simulink library "tqd"  (R2021b)
settings: Solver=VariableStepAuto  StartTime=0.0  StopTime=10.0  RelTol=1e-3
undefined symbols (not defined in the file): ATQD_AfterTqMinGain_X_Deg, ATQD_APSCreepBaseTqD_X_kph, ATQD_APSCreepBaseTqD_Y_Deg, ATQD_APSCreepBaseTqR_X_kph, ATQD_APSCreepBaseTqR_Y_Deg, ATQD_APSCreepIterm_X_kph, ATQD_APSCreepIterm_Y_kph, ATQD_APSCreepPterm_X_kph, ATQD_APSCreepPterm_Y_kph, ATQD_APSDecReq_X_kph, ATQD_APSDecReq_Y_mps2, ATQD_APSDecReqCMD_X_kph, ATQD_APSDecReqTs_X_pct, ATQD_APSDecTimeGain_X_Deg, ATQD_APSDecTimeGain_Y_s, ATQD_APSReqLowSpd_X_Deg, ATQD_AutoHoldReleaseBPS_X_Deg, ATQD_AWDLoadTrqnsGain_X_kg, ATQD_AWDLoadTrqnsGain_Y_pct, ATQD_BOSEnBPSPosn_X_kph, ATQD_BOSMap_X_rpm, ATQD_BOSMap_Y_pct, ATQD_CreepBaseTqD_X_kph, ATQD_CreepBaseTqD_Y_Deg, ATQD_CreepBaseTqR_X_kph, ATQD_CreepBaseTqR_Y_Deg, ATQD_CreepBPSDisPosn_X_Deg, ATQD_CreepBPSDisPosnR_X_Deg, ATQD_CreepBPSEnPosn_X_Deg, ATQD_CreepBPSEnPosnR_X_Deg, ATQD_CreepDeltaTq_X_kph, ATQD_CreepIterm_X_kph, ATQD_CreepIterm_Y_kph, ATQD_CreepItermMaxLimit_X_pct, ATQD_CreepPreloadTime_X_kph, ATQD_CreepPreloadTq_X_kph, ATQD_CreepPreloadTq_Y_s, ATQD_CreepProtTq_X_Deg, ATQD_CreepPterm_X_kph, ATQD_CreepPterm_Y_kph, ATQD_CreepRrTqSpRat_X_rpm, ATQD_CreepRrTqSpRat_Y_Nm, ATQD_CreepTargetSpdD_X_pct, ATQD_CreepTargetSpdR_X_pct, ATQD_ECOTqMapD_X_rpm, ATQD_ECOTqMapD_Y_pct, ATQD_EMTqMapD_X_rpm, ATQD_EMTqMapD_Y_pct, ATQD_EOPDTqMapDCon_X_rpm, ATQD_EOPDTqMapDCon_Y_Deg, ATQD_EscapeModePedTq_X_pct, ATQD_EscapeModePedTq_Y_rpm, ATQD_EscapeModePedTqFr_X_pct, ATQD_EscapeModePedTqFr_Y_rpm, ATQD_EstInitVehWeight_X_c, ATQD_FAfterTqCMDGain_X_rpm, ATQD_FAfterTqCMDGain_Y_pct, ATQD_FrLossMAPLowV_X_rpm, ATQD_FrLossMAPLowV_Y_Nm, ATQD_FrMotActReduce_X_rpm ... (+772)
libraries: simulink x211, hcu_lib x179, tqr x3
(part 1 of 28)
settings Model: Creator=13615  LastModifiedBy=FVT24123
settings SolverCC: AlgebraicLoopSolver=TrustRegion
settings DataIOCC: SaveFormat=Array  SignalLoggingSaveFormat=ModelDataLogs  ReturnWorkspaceOutputs=off
settings OptimizationCC: BlockReduction=off  BooleanDataType=off
settings DebuggingCC: SaveWithParameterizedLinksMsg=none  UnderspecifiedInitializationDetection=Classic  MergeDetectMultiDrivingBlocksExec=none  SignalResolutionControl=TryResolveAllWithWarning
settings HardwareCC: TargetUnknown=on
settings ModelReferenceCC: PropagateSignalLabelsOutOfModel=off
settings SFSimCC: SimUseLocalCustomCode=off
settings RTWCC: RTWUseLocalCustomCode=off
settings ConfigComp: CovMetricSettings=dw  CovSaveCumulativeToWorkspaceVar=on  CovSaveSingleToWorkspaceVar=on

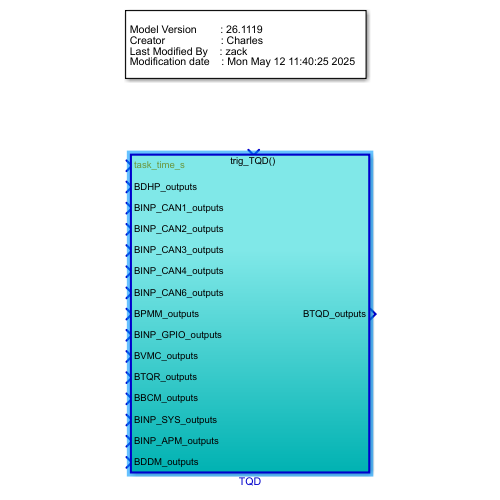
[thumbnail: Simulink's stored preview of the top-level diagram]
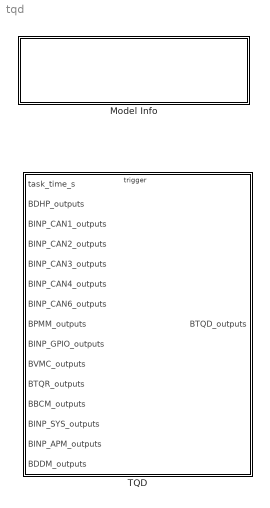
== system tqd ==
  Model Info : Subsystem  LoadFcn=slcm LoadBlock;  InitFcn=slcm('UpdateAllCMBlocksInThisModelInit')  mask(CMBlock){InitialSaveTempField=, InitialBlockCM=None, BlockCM=None, Frame=on, SaveTempField=, DisplayStringWithTags=|, MaskDisplayString=Model Version        : 26.1294\nCreator                   : Charles\nLast Modified By    : FVT24123\nModification date    : Mon Sep 22 17:25:36 2025, HorizontalTextAlignment=Left, LeftAlignmentValue=0.02, SourceBlockDiagram=tqd, TagMaxNumber=20, CMTag1=, CMTag2=, CMTag3=, CMTag4=, CMTag5=, CMTag6=, CMTag7=, CMTag8=, CMTag9=, CMTag10=, CMTag11=, CMTag12=, CMTag13=, CMTag14=, CMTag15=, CMTag16=, CMTag17=, CMTag18=, CMTag19=, CMTag20=}
      mask DisplayStringWithTags=|
      | Model Version        : %<ModelVersion>
      | Creator                   : Charles
      | Last Modified By    : %<LastModifiedBy>
      | Modification date    : %<LastModificationDate>
      mask help: This block allows revision control information to be displayed within the model.
      settings: CopyFcn=slcm CopyBlock;  DeleteFcn=slcm Cancel;  PostSaveFcn=slcm('UpdateAllCMBlocksInThisModel')  NameChangeFcn=slcm Rename;  OpenFcn=slcm
      mask Display: text(str2num(LeftAlignmentValue), 0.5, MaskDisplayString, 'HorizontalAlignment', HorizontalTextAlignment)
  TQD : Subsystem
      settings: RTWSystemCode=Nonreusable function  RTWFcnNameOpts=Use subsystem name  RTWFileNameOpts=Use subsystem name

== system tqd/Model Info ==
  EmptySubsystem : Subsystem

== system tqd/TQD ==
  task_time_s : Inport
  BDHP_outputs : Inport  Port=2  OutDataTypeStr=Bus: BDHP_outputs
  BINP_CAN1_outputs : Inport  Port=3  OutDataTypeStr=Bus: BINP_CAN1_outputs
  BINP_CAN2_outputs : Inport  Port=4  OutDataTypeStr=Bus: BINP_CAN2_outputs
  BINP_CAN3_outputs : Inport  Port=5  OutDataTypeStr=Bus: BINP_CAN3_outputs
  BINP_CAN4_outputs : Inport  Port=6  OutDataTypeStr=Bus: BINP_CAN4_outputs
  BINP_CAN6_outputs : Inport  Port=7  OutDataTypeStr=Bus: BINP_CAN6_outputs
  BPMM_outputs : Inport  Port=8  OutDataTypeStr=Bus: BPMM_outputs
  BINP_GPIO_outputs : Inport  Port=9  OutDataTypeStr=Bus: BINP_GPIO_outputs
  BVMC_outputs : Inport  Port=10  OutDataTypeStr=Bus: BVMC_outputs
  BTQR_outputs : Inport  Port=11  OutDataTypeStr=Bus: BTQR_outputs  LockScale=on
  BBCM_outputs : Inport  Port=12  OutDataTypeStr=Bus: BBCM_outputs
  BINP_SYS_outputs : Inport  Port=13  OutDataTypeStr=Bus: BINP_SYS_outputs
  BINP_APM_outputs : Inport  Port=14  OutDataTypeStr=Bus: BINP_APM_outputs
  BDDM_outputs : Inport  Port=15  OutDataTypeStr=Bus: BDDM_outputs
  trig_TQD : TriggerPort  TriggerType=function-call  VariantControl=(inherit)
  Bus Creator1 : BusCreator  Inputs=118  OutDataTypeStr=Bus: BTQD_outputs  NonVirtualBus=on
  Bus Selector : BusSelector  OutputSignals=VINP_IVIPWModeReq_enum,VINP_IVICreepSWReq_flg,VINP_RollModeSWCmd_enum,VINP_IVIPwrLockSW_enum,VINP_IVIISAOffsetSpd_enum,VINP_Distanceunit_flg,VINP_SmartEcoModeSW_flg,VINP_IVISnowModeCmd_flg,VINP_IVIACCAdaptiveSta_flg,VINP_IVITrailerModeSWSta_flg
  Bus Selector1 : BusSelector  OutputSignals=VDHP_ActAPSPosn_pct,VDHP_LowIdleAccPedal_flg
  Bus Selector10 : BusSelector  OutputSignals=VBCM_BrakeLamp_flg,VBCM_UserNow_enum
  Bus Selector11 : BusSelector  OutputSignals=VINP_FlashRegenMode_enum,VINP_VehicleType_enum,VINP_SWCType_enum
  Bus Selector12 : BusSelector  OutputSignals=VINP_CAASSta_enum,VINP_APSStaSystem_enum
  Bus Selector13 : BusSelector  OutputSignals=VINP_FrEDURotateDirction_enum,VINP_RrEDURotateDirction_enum,VINP_FrTMSpd_rpm,VINP_RrTMSpd_rpm,VINP_FrRegenAvailTq_Nm,VINP_RrRegenAvailTq_Nm,VINP_FrEDURealTMTq_Nm,VINP_RrEDURealTMTq_Nm,VINP_FrMotorAvailTq_Nm,VINP_RrMotorAvailTq_Nm,VINP_MCUWarnF_enum,VINP_MCUWarnR_enum,VINP_FrMCUDCBusVolt_V,VINP_RrMCUDCBusVolt_V,VINP_FrMCUTemp_C,VINP_FrTMTemp_C,VINP_RrMCUTemp_C,VINP_RrTMTemp_C
  Bus Selector14 : BusSelector  OutputSignals=VINP_SWCRegenUp_flg,VINP_SWCRegenDown_flg
  Bus Selector15 : BusSelector  OutputSignals=VDDM_VCURAPSErrLv2_flg,VDDM_VCURAPSErrLv3_flg,VDDM_EPBSigErrCFS_flg,VDDM_EPB1Err_flg,VDDM_ESC1Err_flg,VDDM_ESC5Err_flg,VDDM_LimpHomeAct_flg,VDDM_VehMalfunLevel_enum,VDDM_Shifter1Err_flg,VDDM_ShifterSigErrCFS_flg,VDDM_MCUF1Err_flg,VDDM_MCUR1Err_flg,VDDM_RegenErrCFS_flg,VDDM_4D2CErr_flg
  Bus Selector2 : BusSelector  OutputSignals=VINP_VehSpeed_kph,VINP_BrkSwSta_flg,VINP_BrkSwV_flg,VINP_BrkPedalPos_pct,VINP_BrkPedalPosSta_flg,VINP_FrPTCSActive_flg,VINP_RrPTCSActive_flg,VINP_FrntAxlTrqReqDrv_Nm,VINP_RearAxlTrqReqDrv_Nm,VINP_FrRBCActive_flg,VINP_RrRBCActive_flg,VINP_FrntAxlTrqReqBrk_Nm,VINP_RearAxlTrqReqBrk_Nm,VINP_CrashOutputSts_enum,VINP_LongAccel_Gps,VINP_EPBCarWashMode_flg,VINP_EPBErrSta_enum,VINP_EPBSta_enum,VINP_DOASta_flg,VINP_GRADE_Deg,VINP_HSAActive_flg,VINP_DriverSeatBeltCmd_flg,VINP_AVHActive_flg,VINP_PsngrSeatBeltCmd_flg,VINP_RDriverSeatBeltCmd_flg,VINP_RCenterSeatBeltCmd_flg,VINP_RPsngrSeatBeltCmd_flg,VINP_YawRate_degps,VINP_SASAngle_Deg,VINP_ESCActive_flg,VINP_ABSActive_flg,VINP_LFRawWhlSpeed_kph,VINP_LRRawWhlSpeed_kph,VINP_RFRawWhlSpeed_kph,VINP_RRRawWhlSpeed_kph,VINP_ESCOFFStatus_enum
  Bus Selector3 : BusSelector  OutputSignals=VINP_BrakeSWGPIO_flg,VINP_CrashSignalGPIO_flg,VINP_DrDoorSW_flg,VINP_SeatSW_flg,VINP_HoodSW_flg,VINP_TailgateSW_flg,VINP_PsDoorSW_flg,VINP_RRDoorSW_flg,VINP_RLDoorSW_flg
  Bus Selector4 : BusSelector  OutputSignals=VINP_ShifterHandleCmd_enum,VINP_HVBPwrAvailDchrg_kW,VINP_HVBPwrAvailChrg_kW,VINP_HVBattErr_flg,VINP_DCDCFaultSta_enum,VINP_ChrgPlugSta_enum,VINP_HVBattSOC_pct,VINP_HVBattSOCDis_pct,VINP_HVBMTempMax_C,VINP_HVBMTempMin_C,VINP_ShifterFailsta_enum
  Bus Selector5 : BusSelector  OutputSignals=VVMC_ADASForceIdle_flg,VVMC_ACCRequiredAccel_mps2,VVMC_ACCVehHoldReq_flg,VVMC_ADASActive_flg,VVMC_ADASWhlTqReq_Nm,VVMC_CruzActive_flg,VVMC_CruzWhlTqReq_Nm,VVMC_MSAActive_flg,VVMC_MSAWhlTqReq_Nm,VVMC_APSActive_flg,VVMC_APSSpeedCMD_kph,VVMC_APSShiftPosnReq_enum,VVMC_ACCPedalOvrd_flg,VVMC_LongAcc_Gps,VVMC_ActMaxSlideRate_pct,VVMC_EstSlope_Deg,VVMC_APSReq_enum,VVMC_RWDRDCActive_enum,VVMC_ActLRSlideRate_pct,VVMC_ActRRSlideRate_pct,VVMC_ActStESCYaw_Dps,VVMC_CCCtrlSta_enum,VVMC_MSACtrlSta_enum,VVMC_LVDAACCStatusInformation_flg,VVMC_ACCObjDist_m,VVMC_MeterIndSpeed_raw32,VVMC_RearTqRatio_rat,VVMC_CalibratedGyroY_Dps,VVMC_CAASActive_flg,VVMC_SetACCDisableAPS_flg
  Bus Selector6 : BusSelector  OutputSignals=VINP_SWCResUpSta_flg,VINP_SWCSetdownSta_flg,VINP_SWCACCSta_flg,VINP_SWCCANCELSta_flg,VINP_SWC2LScrollUpSta_flg,VINP_SWC2LScrollDownSta_flg,VINP_SWC2LScrollPressSta_flg,VINP_SWC2LADASSta_flg,VINP_SWC2RScrollPressSta_flg,VINP_SWC2RScrollUpSta_flg,VINP_SWC2RScrollDownSta_flg,VINP_SWC2LDriveModeSta_flg,VINP_SWC2RRightSta_flg,VINP_SWC2RLeftSta_flg,VINP_SWC2RCustomizeSta_flg
  Bus Selector7 : BusSelector  OutputSignals=VPMM_PowerSta_enum,VPMM_DrivetrainSelect_enum,VPMM_SysPowerMode_enum
  Bus Selector8 : BusSelector  OutputSignals=VTQR_ActualFEDUWhlTqReq_Nm,VTQR_ActualREDUWhlTqReq_Nm,VTQR_NoABSFEDUWhlTqReq_Nm,VTQR_NoABSREDUWhlTqReq_Nm,VTQR_RShaftSpdTqLimLow_flg,VTQR_RTimerTqLimLow_flg,VTQR_FShaftSpdTqLimLow_flg,VTQR_FTimerTqLimLow_flg,VTQR_FrFirstOrderInpTs_c,VTQR_RrFirstOrderInpTs_c,VTQR_FrRateLimitInc_Nm,VTQR_FrRateLimitDec_Nm,VTQR_RrRateLimitInc_Nm,VTQR_RrRateLimitDec_Nm,VTQR_FrTqZeroTransLowBound_Nm,VTQR_RrTqZeroTransUpBound_Nm
  Bus Selector9 : BusSelector  OutputSignals=VINP_ADASISASta_enum,VINP_ADASVehSpdLim_enum,VINP_ADASACCSta_enum,VINP_ADASSLIFSpdLim_enum,VINP_ADASAEBSta_enum
  Constant2 : Constant  Value=KTQD_IVIEscapeModeCmd_flg
  Constant4 : Constant  Value=KTQD_BCMUserNowSetting_enum
  Ground1 : Ground
  SWC_HandShake : Subsystem
  Subsystem : Subsystem
  TorqueDemand : Subsystem
  BTQD_outputs : Outport  OutDataTypeStr=Bus: BTQD_outputs
  wires:
  Bus Selector2/19 -> TorqueDemand/25(VINP_DOASta_flg)  "<VINP_DOASta_flg>"
  Bus Selector2/18 -> TorqueDemand/24(VINP_EPBSta_enum)  "<VINP_EPBSta_enum>"
  Bus Selector2/17 -> TorqueDemand/23(VINP_EPBErrSta_enum)  "<VINP_EPBErrSta_enum>"
  Bus Selector2/16 -> TorqueDemand/22(VINP_EPBCarWashMode_flg)  "<VINP_EPBCarWashMode_flg>"
  Bus Selector8/2 -> TorqueDemand/139(VTQR_ActualREDUWhlTqReq_Nm)  "<VTQR_ActualREDUWhlTqReq_Nm>"
  Bus Selector2/15 -> TorqueDemand/21(VINP_LongAccel_Gps)  "<VINP_LongAccel_Gps>"
  Bus Selector8/1 -> TorqueDemand/138(VTQR_ActualFEDUWhlTqReq_Nm)  "<VTQR_ActualFEDUWhlTqReq_Nm>"
  Bus Selector5/6 -> TorqueDemand/104(VVMC_CruzActive_flg)  "<VVMC_CruzActive_flg>"
  BTQR_outputs/1 -> Bus Selector8/1
  Bus Selector3/2 -> TorqueDemand/130(VINP_CrashSignalGPIO_flg)  "<VINP_CrashSignalGPIO_flg>"
  Bus Selector3/1 -> TorqueDemand/129(VINP_BrakeSWGPIO_flg)  "<VINP_BrakeSWGPIO_flg>"
  Bus Selector5/9 -> TorqueDemand/107(VVMC_MSAWhlTqReq_Nm)  "<VVMC_MSAWhlTqReq_Nm>"
  Bus Selector5/4 -> TorqueDemand/102(VVMC_ADASActive_flg)  "<VVMC_ADASActive_flg>"
  Bus Selector5/8 -> TorqueDemand/106(VVMC_MSAActive_flg)  "<VVMC_MSAActive_flg>"
  Bus Selector5/7 -> TorqueDemand/105(VVMC_CruzWhlTqReq_Nm)  "<VVMC_CruzWhlTqReq_Nm>"
  Bus Selector5/5 -> TorqueDemand/103(VVMC_ADASWhlTqReq_Nm)  "<VVMC_ADASWhlTqReq_Nm>"
  Bus Selector2/14 -> TorqueDemand/20(VINP_CrashOutputSts_enum)  "<VINP_CrashOutputSts_enum>"
  BDHP_outputs/1 -> Bus Selector1/1
  Bus Selector2/5 -> TorqueDemand/11(VINP_BrkPedalPosSta_flg)  "<VINP_BrkPedalPosSta_flg>"
  Bus Selector/1 -> TorqueDemand/43(VINP_IVIPWModeReq_enum)  "<VINP_IVIPWModeReq_enum>"
  [BINP_CAN4_outputs] -> Bus Selector6/1  "BINP_CAN4_outputs"
  BINP_CAN2_outputs/1 -> Bus Selector/1  "BINP_CAN2_outputs"
  Ground1/1 -> TorqueDemand/154(VINP_PBWMotorPos_enum)
  BVMC_outputs/1 -> Bus Selector5/1
  Bus Selector2/11 -> TorqueDemand/17(VINP_RrRBCActive_flg)  "<VINP_RrRBCActive_flg>"
  Bus Selector2/7 -> TorqueDemand/13(VINP_RrPTCSActive_flg)  "<VINP_RrPTCSActive_flg>"
  Bus Selector7/2 -> TorqueDemand/5(VPMM_DrivetrainSelect_enum)  "<VPMM_DrivetrainSelect_enum>"
  BINP_GPIO_outputs/1 -> Bus Selector3/1
  Bus Selector1/2 -> TorqueDemand/3(VDHP_LowIdleAccPedal_flg)  "<VDHP_LowIdleAccPedal_flg>"
  Bus Selector1/1 -> TorqueDemand/2(VDHP_ActAPSPosn_pct)  "<VDHP_ActAPSPosn_pct>"
  Bus Selector2/10 -> TorqueDemand/16(VINP_FrRBCActive_flg)  "<VINP_FrRBCActive_flg>"
  Bus Selector2/9 -> TorqueDemand/15(VINP_RearAxlTrqReqDrv_Nm)  "<VINP_RearAxlTrqReqDrv_Nm>"
  Bus Selector2/8 -> TorqueDemand/14(VINP_FrntAxlTrqReqDrv_Nm)  "<VINP_FrntAxlTrqReqDrv_Nm>"
  Bus Selector2/13 -> TorqueDemand/19(VINP_RearAxlTrqReqBrk_Nm)  "<VINP_RearAxlTrqReqBrk_Nm>"
  Bus Selector2/12 -> TorqueDemand/18(VINP_FrntAxlTrqReqBrk_Nm)  "<VINP_FrntAxlTrqReqBrk_Nm>"
  Bus Selector2/4 -> TorqueDemand/10(VINP_BrkPedalPos_pct)  "<VINP_BrkPedalPos_pct>"
  Bus Selector2/3 -> TorqueDemand/9(VINP_BrkSwV_flg)  "<VINP_BrkSwV_flg>"
  Bus Selector2/2 -> TorqueDemand/8(VINP_BrkSwSta_flg)  "<VINP_BrkSwSta_flg>"
  Bus Selector2/1 -> TorqueDemand/7(VINP_VehSpeed_kph)  "<VINP_VehSpeed_kph>"
  Bus Selector2/6 -> TorqueDemand/12(VINP_FrPTCSActive_flg)  "<VINP_FrPTCSActive_flg>"
  Bus Selector7/1 -> TorqueDemand/4(VPMM_PowerSta_enum)  "<VPMM_PowerSta_enum>"
  task_time_s/1 -> TorqueDemand/1(task_time_s)  "task_time_s"
  BINP_CAN1_outputs/1 -> Bus Selector2/1
  BPMM_outputs/1 -> Bus Selector7/1
  Bus Creator1/1 -> BTQD_outputs/1  "BTQD_outputs"
  Bus Selector2/20 -> TorqueDemand/26(VINP_GRADE_Deg)  "<VINP_GRADE_Deg>"
  Bus Selector2/21 -> TorqueDemand/27(VINP_HSAActive_flg)  "<VINP_HSAActive_flg>"
  Bus Selector/2 -> TorqueDemand/44(VINP_IVICreepSWReq_flg)  "<VINP_IVICreepSWReq_flg>"
  Bus Selector2/22 -> TorqueDemand/28(VINP_DriverSeatBeltCmd_flg)  "<VINP_DriverSeatBeltCmd_flg>"
  Bus Selector3/3 -> TorqueDemand/131(VINP_DrDoorSW_flg)  "<VINP_DrDoorSW_flg>"
  Bus Selector3/4 -> TorqueDemand/132(VINP_SeatSW_flg)  "<VINP_SeatSW_flg>"
  Bus Selector7/3 -> TorqueDemand/6(VPMM_SysPowerMode_enum)  "<VPMM_SysPowerMode_enum>"
  Bus Selector8/3 -> TorqueDemand/140(VTQR_NoABSFEDUWhlTqReq_Nm)  "<VTQR_NoABSFEDUWhlTqReq_Nm>"
  Bus Selector8/4 -> TorqueDemand/141(VTQR_NoABSREDUWhlTqReq_Nm)  "<VTQR_NoABSREDUWhlTqReq_Nm>"
  Bus Selector2/23 -> TorqueDemand/29(VINP_AVHActive_flg)  "<VINP_AVHActive_flg>"
  Bus Selector5/10 -> TorqueDemand/108(VVMC_APSActive_flg)  "<VVMC_APSActive_flg>"
  Bus Selector5/11 -> TorqueDemand/109(VVMC_APSSpeedCMD_kph)  "<VVMC_APSSpeedCMD_kph>"
  Bus Selector5/12 -> TorqueDemand/110(VVMC_APSShiftPosnReq_enum)  "<VVMC_APSShiftPosnReq_enum>"
  Bus Selector5/13 -> TorqueDemand/111(VVMC_ACCPedalOvrd_flg)  "<VVMC_ACCPedalOvrd_flg>"
  Bus Selector2/24 -> TorqueDemand/30(VINP_PsngrSeatBeltCmd_flg)  "<VINP_PsngrSeatBeltCmd_flg>"
  Bus Selector2/25 -> TorqueDemand/31(VINP_RDriverSeatBeltCmd_flg)  "<VINP_RDriverSeatBeltCmd_flg>"
  Bus Selector2/27 -> TorqueDemand/33(VINP_RPsngrSeatBeltCmd_flg)  "<VINP_RPsngrSeatBeltCmd_flg>"
  Bus Selector/3 -> TorqueDemand/45(VINP_RollModeSWCmd_enum)  "<VINP_RollModeSWCmd_enum>"
  Bus Selector5/14 -> TorqueDemand/112(VVMC_LongAcc_Gps)  "<VVMC_LongAcc_Gps>"
  Bus Selector5/15 -> TorqueDemand/113(VVMC_ActMaxSlideRate_pct)  "<VVMC_ActMaxSlideRate_pct>"
  Bus Selector5/17 -> TorqueDemand/115(VVMC_APSReq_enum)  "<VVMC_APSReq_enum>"
  Bus Selector5/16 -> TorqueDemand/114(VVMC_EstSlope_Deg)  "<VVMC_EstSlope_Deg>"
  Bus Selector2/26 -> TorqueDemand/32(VINP_RCenterSeatBeltCmd_flg)  "<VINP_RCenterSeatBeltCmd_flg>"
  Bus Selector3/5 -> TorqueDemand/133(VINP_HoodSW_flg)  "<VINP_HoodSW_flg>"
  Bus Selector3/6 -> TorqueDemand/134(VINP_TailgateSW_flg)  "<VINP_TailgateSW_flg>"
  Bus Selector3/7 -> TorqueDemand/135(VINP_PsDoorSW_flg)  "<VINP_PsDoorSW_flg>"
  Bus Selector3/8 -> TorqueDemand/136(VINP_RRDoorSW_flg)  "<VINP_RRDoorSW_flg>"
  Bus Selector3/9 -> TorqueDemand/137(VINP_RLDoorSW_flg)  "<VINP_RLDoorSW_flg>"
  Bus Selector6/1 -> TorqueDemand/82(VINP_SWCResUpSta_flg)  "<VINP_SWCResUpSta_flg>"
  Bus Selector/4 -> TorqueDemand/46(VINP_IVIPwrLockSW_enum)  "<VINP_IVIPwrLockSW_enum>"
  Bus Selector5/18 -> TorqueDemand/116(VVMC_RWDRDCActive_enum)  "<VVMC_RWDRDCActive_enum>"
  Bus Selector5/19 -> TorqueDemand/117(VVMC_ActLRSlideRate_pct)  "<VVMC_ActLRSlideRate_pct>"
  Bus Selector5/20 -> TorqueDemand/118(VVMC_ActRRSlideRate_pct)  "<VVMC_ActRRSlideRate_pct>"
  Bus Selector5/21 -> TorqueDemand/119(VVMC_ActStESCYaw_degps)  "<VVMC_ActStESCYaw_Dps>"
  Bus Selector2/28 -> TorqueDemand/34(VINP_YawRate_degps)  "<VINP_YawRate_degps>"
  Bus Selector2/29 -> TorqueDemand/35(VINP_SASAngle_Deg)  "<VINP_SASAngle_Deg>"
  TorqueDemand/24(VTQD_DriverWhlTqDemRr_Nm) -> Bus Creator1/24
  TorqueDemand/25(VTQD_FrEDUActTq_Nm) -> Bus Creator1/25
  TorqueDemand/26(VTQD_RrEDUActTq_Nm) -> Bus Creator1/26
  TorqueDemand/27(VTQD_FrEDURolRgnTq_Nm) -> Bus Creator1/27
  TorqueDemand/28(VTQD_RrEDURolRgnTq_Nm) -> Bus Creator1/28
  TorqueDemand/29(VTQD_FrEDUSpd_rpm) -> Bus Creator1/29
  TorqueDemand/30(VTQD_RrEDUSpd_rpm) -> Bus Creator1/30
  TorqueDemand/42(VTQD_FrUdcMin_V) -> Bus Creator1/42
  TorqueDemand/43(VTQD_FrUdcMax_V) -> Bus Creator1/43
  TorqueDemand/44(VTQD_RrIdcMin_A) -> Bus Creator1/44
  TorqueDemand/45(VTQD_RrIdcMax_A) -> Bus Creator1/45
  TorqueDemand/46(VTQD_RrUdcMin_V) -> Bus Creator1/46
  TorqueDemand/47(VTQD_RrUdcMax_V) -> Bus Creator1/47
  TorqueDemand/48(VTQD_CoordWhlTqDemFr_Nm) -> Bus Creator1/48
  TorqueDemand/49(VTQD_CoordWhlTqDemRr_Nm) -> Bus Creator1/49
  TorqueDemand/50(VTQD_CreepEnable_flg) -> Bus Creator1/50
  TorqueDemand/51(VTQD_CrashDetd_flg) -> Bus Creator1/51
  TorqueDemand/52(VTQD_DiagHCrash_flg) -> Bus Creator1/52
  TorqueDemand/53(VTQD_ReBrakeLPReq_flg) -> Bus Creator1/53
  TorqueDemand/54(VTQD_LoSpdBrkCtrl_flg) -> Bus Creator1/54
  TorqueDemand/55(VTQD_LowIdleAccPedal_flg) -> Bus Creator1/55
  TorqueDemand/56(VTQD_APSStaSys_enum) -> Bus Creator1/56
  TorqueDemand/57(VTQD_APSReq_enum) -> Bus Creator1/57
  TorqueDemand/58(VTQD_APSDecReqA_flg) -> Bus Creator1/58
  TorqueDemand/59(VTQD_APSDecReq_mps2) -> Bus Creator1/59
  TorqueDemand/60(VTQD_ExtShftAllow_flg) -> Bus Creator1/60
  TorqueDemand/61(VTQD_EstVehWeightResult_kg) -> Bus Creator1/61
  TorqueDemand/62(VTQD_BOSEnable_flg) -> Bus Creator1/62
  TorqueDemand/63(VTQD_CreepON_flg) -> Bus Creator1/63
  TorqueDemand/64(VTQD_PreLoadHold_flg) -> Bus Creator1/64
  TorqueDemand/65(VTQD_PreLoadPreEn_flg) -> Bus Creator1/65
  TorqueDemand/66(VTQD_CreepPrLoadEnable_flg) -> Bus Creator1/66
  TorqueDemand/67(VTQD_RDCActive_enum) -> Bus Creator1/67
  TorqueDemand/68(VTQD_EquivAccPedalSWSta_flg) -> Bus Creator1/68
  TorqueDemand/69(VTQD_DriveProtEn_flg) -> Bus Creator1/69
  TorqueDemand/70(VTQD_ActParkRequest_flg) -> Bus Creator1/70
  TorqueDemand/71(VTQD_RegenTqLimitEn_flg) -> Bus Creator1/71
  Bus Selector5/1 -> TorqueDemand/99(VINP_ADASForceIdle_flg)  "<VVMC_ADASForceIdle_flg>"
  Bus Selector5/2 -> TorqueDemand/100(VVMC_ACCRequiredAccel_mps2)  "<VVMC_ACCRequiredAccel_mps2>"
  Bus Selector5/3 -> TorqueDemand/101(VINP_ACCVehHoldReq_flg)  "<VVMC_ACCVehHoldReq_flg>"
  TorqueDemand/72(VTQD_PedAccTqEn_flg) -> Bus Creator1/72
  TorqueDemand/73(VTQD_IVIPwrLockSta_enum) -> Bus Creator1/73
  TorqueDemand/74(VTQD_ExtDoorAllow_flg) -> Bus Creator1/74
  TorqueDemand/75(VTQD_WhlTqCapGenFr_Nm) -> Bus Creator1/75
  TorqueDemand/76(VTQD_WhlTqCapGenRr_Nm) -> Bus Creator1/76
  TorqueDemand/77(VTQD_OPDHoldLamp_flg) -> Bus Creator1/77
  TorqueDemand/78(VTQD_RegenMode_enum) -> Bus Creator1/78
  BINP_CAN6_outputs/1 -> Bus Selector9/1
  Bus Selector9/1 -> TorqueDemand/157(VINP_ADASISASta_enum)  "<VINP_ADASISASta_enum>"
  Bus Selector9/2 -> TorqueDemand/158(VINP_ADASVehSpdLim_kph)  "<VINP_ADASVehSpdLim_enum>"
  Bus Selector5/22 -> TorqueDemand/120(VVMC_CCCtrlSta_enum)  "<VVMC_CCCtrlSta_enum>"
  Bus Selector5/23 -> TorqueDemand/121(VVMC_MSACtrlSta_enum)  "<VVMC_MSACtrlSta_enum>"
  Bus Selector/5 -> TorqueDemand/47(VINP_IVIISAOffsetSpd_enum)  "<VINP_IVIISAOffsetSpd_enum>"
  BBCM_outputs/1 -> Bus Selector10/1
  Bus Selector10/1 -> TorqueDemand/155(VBCM_BrakeLamp_flg)  "<VBCM_BrakeLamp_flg>"
  Bus Selector6/2 -> TorqueDemand/83(VINP_SWCSetdownSta_flg)  "<VINP_SWCSetdownSta_flg>"
  Bus Selector6/3 -> TorqueDemand/84(VINP_SWCACCSta_flg)  "<VINP_SWCACCSta_flg>"
  Bus Selector6/4 -> TorqueDemand/85(VINP_SWCCANCELSta_flg)  "<VINP_SWCCANCELSta_flg>"
  TorqueDemand/79(VTQD_SaveRegenMode_enum) -> Bus Creator1/79
  TorqueDemand/80(VTQD_FDCVCURegenMode_enum) -> Bus Creator1/80
  TorqueDemand/81(VTQD_SpdCtrlMode_enum) -> Bus Creator1/81
  TorqueDemand/82(VTQD_SpdCtrlSta_flg) -> Bus Creator1/82
  TorqueDemand/83(VTQD_SetSpd_kph) -> Bus Creator1/83
  BINP_SYS_outputs/1 -> Bus Selector11/1
  Bus Selector11/1 -> TorqueDemand/162(VINP_FlashRegenMode_enum)  "<VINP_FlashRegenMode_enum>"
  Bus Selector9/3 -> TorqueDemand/159(VINP_ADASACCSta_enum)  "<VINP_ADASACCSta_enum>"
  Bus Selector5/24 -> TorqueDemand/122(VVMC_LVDAACCStatusInformation_flg)  "<VVMC_LVDAACCStatusInformation_flg>"
  Bus Selector5/25 -> TorqueDemand/123(VVMC_ACCObjDist_m)  "<VVMC_ACCObjDist_m>"
  Bus Selector5/26 -> TorqueDemand/124(VVMC_MeterIndSpeed_raw32)  "<VVMC_MeterIndSpeed_raw32>"
  TorqueDemand/84(VTQD_SWCCancelSta_flg) -> Bus Creator1/84
  TorqueDemand/85(VTQD_SWCSetdownSta_flg) -> Bus Creator1/85
  TorqueDemand/86(VTQD_SWCResUpSta_flg) -> Bus Creator1/86
  Bus Selector/6 -> TorqueDemand/48(VINP_Distanceunit_flg)  "<VINP_Distanceunit_flg>"
  Bus Selector5/27 -> TorqueDemand/125(VVMC_RearTqRatio_rat)  "<VVMC_RearTqRatio_rat>"
  TorqueDemand/87(VTQD_CreepBaseTqD_Nm) -> Bus Creator1/87
  Bus Selector5/29 -> TorqueDemand/127(VVMC_CAASActive_flg)  "<VVMC_CAASActive_flg>"
  Bus Selector5/28 -> TorqueDemand/126(VVMC_CalibratedGyroY_Dps)  "<VVMC_CalibratedGyroY_Dps>"
  TorqueDemand/88(VTQD_VehActSpd_kph) -> Bus Creator1/88
  TorqueDemand/89(VTQD_RegenLimIndSta_flg) -> Bus Creator1/89
  Bus Selector/7 -> TorqueDemand/49(VINP_SmartEcoModeSW_flg)  "<VINP_SmartEcoModeSW_flg>"
  Bus Selector2/30 -> TorqueDemand/36(VINP_ESCActive_flg)  "<VINP_ESCActive_flg>"
  Bus Selector2/31 -> TorqueDemand/37(VINP_ABSActive_flg)  "<VINP_ABSActive_flg>"
  BINP_APM_outputs/1 -> Bus Selector12/1
  Bus Selector12/1 -> TorqueDemand/165(VINP_CAASSta_enum)  "<VINP_CAASSta_enum>"
  TorqueDemand/90(VTQD_BrkSwSta_flg) -> Bus Creator1/90
  Bus Selector4/1 -> TorqueDemand/53(VINP_ShifterHandleCmd_enum)  "<VINP_ShifterHandleCmd_enum>"
  Bus Selector4/2 -> TorqueDemand/54(VINP_HVBPwrAvailDchrg_kw)  "<VINP_HVBPwrAvailDchrg_kW>"
  Bus Selector4/3 -> TorqueDemand/55(VINP_HVBPwrAvailChrg_kw)  "<VINP_HVBPwrAvailChrg_kW>"
  Bus Selector4/4 -> TorqueDemand/56(VINP_HVBattErr_flg)  "<VINP_HVBattErr_flg>"
  Bus Selector4/5 -> TorqueDemand/57(VINP_DCDCFaultSta_enum)  "<VINP_DCDCFaultSta_enum>"
  Bus Selector4/6 -> TorqueDemand/58(VINP_ChrgPlugSta_enum)  "<VINP_ChrgPlugSta_enum>"
  Bus Selector4/7 -> TorqueDemand/59(VINP_HVBattSOC_pct)  "<VINP_HVBattSOC_pct>"
  Bus Selector4/8 -> TorqueDemand/60(VINP_HVBattSOCDis_pct)  "<VINP_HVBattSOCDis_pct>"
  Bus Selector4/9 -> TorqueDemand/61(VINP_HVBMTempMax_C)  "<VINP_HVBMTempMax_C>"
  Bus Selector4/10 -> TorqueDemand/62(VINP_HVBMTempMin_C)  "<VINP_HVBMTempMin_C>"
  Bus Selector13/1 -> TorqueDemand/64(VINP_FrEDURotateDirction_enum)  "<VINP_FrEDURotateDirction_enum>"
  Bus Selector13/2 -> TorqueDemand/65(VINP_RrEDURotateDirction_enum)  "<VINP_RrEDURotateDirction_enum>"
  Bus Selector13/3 -> TorqueDemand/66(VINP_FrTMSpd_RPM)  "<VINP_FrTMSpd_rpm>"
  Bus Selector13/4 -> TorqueDemand/67(VINP_RrTMSpd_RPM)  "<VINP_RrTMSpd_rpm>"
  Bus Selector13/5 -> TorqueDemand/68(VINP_FrRegenAvailTq_Nm)  "<VINP_FrRegenAvailTq_Nm>"
  Bus Selector13/6 -> TorqueDemand/69(VINP_RrRegenAvailTq_Nm)  "<VINP_RrRegenAvailTq_Nm>"
  Bus Selector13/9 -> TorqueDemand/72(VINP_FrMotorAvailTq_Nm)  "<VINP_FrMotorAvailTq_Nm>"
  Bus Selector13/10 -> TorqueDemand/73(VINP_RrMotorAvailTq_Nm)  "<VINP_RrMotorAvailTq_Nm>"
  Bus Selector13/11 -> TorqueDemand/74(VINP_MCUWarnF_enum)  "<VINP_MCUWarnF_enum>"
  Bus Selector13/12 -> TorqueDemand/75(VINP_MCUWarnR_enum)  "<VINP_MCUWarnR_enum>"
  [BTQD_CAN3MCU_outputs] -> Bus Selector13/1
  [BINP_CAN3_outputs] -> Bus Selector4/1
  BINP_CAN3_outputs/1 -> [BINP_CAN3_outputs]
  Subsystem/1(BTQD_CAN3MCU_outputs) -> [BTQD_CAN3MCU_outputs]
  [BINP_CAN3_outputs] -> Subsystem/1(BINP_CAN3_outputs)
  Bus Selector13/7 -> TorqueDemand/70(VINP_FrEDURealTMTq_Nm)  "<VINP_FrEDURealTMTq_Nm>"
  Bus Selector13/8 -> TorqueDemand/71(VINP_RrEDURealTMTq_Nm)  "<VINP_RrEDURealTMTq_Nm>"
  BINP_CAN4_outputs/1 -> [BINP_CAN4_outputs]  "BINP_CAN4_outputs"
  [BINP_CAN4_outputs] -> SWC_HandShake/1(In1)
  SWC_HandShake/1(BTQD_CAN4SWC_outputs) -> [BTQD_CAN4SWC_outputs]  "BTQD_CAN4SWC_outputs"
  [BTQD_CAN4SWC_outputs] -> Bus Selector14/1
  Bus Selector14/1 -> TorqueDemand/97(VINP_SWCRegenUp_flg)  "<VINP_SWCRegenUp_flg>"
  Bus Selector14/2 -> TorqueDemand/98(VINP_SWCRegenDown_flg)  "<VINP_SWCRegenDown_flg>"
  Bus Selector5/30 -> TorqueDemand/128(VVMC_SetACCDisableAPS_flg)  "<VVMC_SetACCDisableAPS_flg>"
  TorqueDemand/91(VTQD_SWC2CancelSta_flg) -> Bus Creator1/91
  TorqueDemand/92(VTQD_SWC2SetdownSta_flg) -> Bus Creator1/92
  TorqueDemand/93(VTQD_SWC2ResUpSta_flg) -> Bus Creator1/93
  TorqueDemand/94(VTQD_SWC2LADASSta_flg) -> Bus Creator1/94
  TorqueDemand/95(VTQD_SpdLim4SetSpd_raw32) -> Bus Creator1/95
  TorqueDemand/96(VTQD_SetSpdLimWarn_flg) -> Bus Creator1/96
  Bus Selector/8 -> TorqueDemand/50(VINP_IVISnowModeCmd_flg)  "<VINP_IVISnowModeCmd_flg>"
  Bus Selector6/5 -> TorqueDemand/86(VINP_SWC2LScrollUpSta_flg)  "<VINP_SWC2LScrollUpSta_flg>"
  Bus Selector6/6 -> TorqueDemand/87(VINP_SWC2LScrollDownSta_flg)  "<VINP_SWC2LScrollDownSta_flg>"
  Bus Selector6/7 -> TorqueDemand/88(VINP_SWC2LScrollPressSta_flg)  "<VINP_SWC2LScrollPressSta_flg>"
  Bus Selector6/8 -> TorqueDemand/89(VINP_SWC2LADASSta_flg)  "<VINP_SWC2LADASSta_flg>"
  Bus Selector9/4 -> TorqueDemand/160(VINP_ADASSLIFSpdLim_enum)  "<VINP_ADASSLIFSpdLim_enum>"
  Bus Selector11/2 -> TorqueDemand/163(VINP_VehicleType_enum)  "<VINP_VehicleType_enum>"
  Bus Selector11/3 -> TorqueDemand/164(VINP_SWCType_enum)  "<VINP_SWCType_enum>"
  Bus Selector/9 -> TorqueDemand/51(VINP_IVIACCAdaptiveSta_flg)  "<VINP_IVIACCAdaptiveSta_flg>"
  Bus Selector2/32 -> TorqueDemand/38(VINP_LFRawWhlSpeed_kph)  "<VINP_LFRawWhlSpeed_kph>"
  Bus Selector2/33 -> TorqueDemand/39(VINP_LRRawWhlSpeed_kph)  "<VINP_LRRawWhlSpeed_kph>"
  Bus Selector2/34 -> TorqueDemand/40(VINP_RFRawWhlSpeed_kph)  "<VINP_RFRawWhlSpeed_kph>"
  Bus Selector2/35 -> TorqueDemand/41(VINP_RRRawWhlSpeed_kph)  "<VINP_RRRawWhlSpeed_kph>"
  Bus Selector/10 -> TorqueDemand/52(VINP_IVITrailerModeSWSta_flg)  "<VINP_IVITrailerModeSWSta_flg>"
  Bus Selector10/2 -> TorqueDemand/156(VBCM_UserNow_enum)  "<VBCM_UserNow_enum>"
  Constant4/1 -> TorqueDemand/167(VBCM_RegenModeUserSetting_enum)  "VTQD_BCMUserNowSetting_enum"
  Bus Selector6/9 -> TorqueDemand/90(VINP_SWC2RScrollPressSta_flg)  "<VINP_SWC2RScrollPressSta_flg>"
  Bus Selector6/10 -> TorqueDemand/91(VINP_SWC2RScrollUpSta_flg)  "<VINP_SWC2RScrollUpSta_flg>"
  Bus Selector6/11 -> TorqueDemand/92(VINP_SWC2RScrollDownSta_flg)  "<VINP_SWC2RScrollDownSta_flg>"
  Bus Selector6/12 -> TorqueDemand/93(VINP_SWC2LDriveModeSta_flg)  "<VINP_SWC2LDriveModeSta_flg>"
  Bus Selector6/13 -> TorqueDemand/94(VINP_SWC2RRightSta_flg)  "<VINP_SWC2RRightSta_flg>"
  Bus Selector6/14 -> TorqueDemand/95(VINP_SWC2RLeftSta_flg)  "<VINP_SWC2RLeftSta_flg>"
  Constant2/1 -> TorqueDemand/168(VINP_IVIEscapeModeCmd_flg)  "VTQD_IVIEscapeModeCmd_flg"
  TorqueDemand/97(VTQD_MaxWhlSlideRate_pct) -> Bus Creator1/97
  TorqueDemand/98(VTQD_MinWhlSlideRate_pct) -> Bus Creator1/98
  TorqueDemand/99(VTQD_LeftSlideRate_pct) -> Bus Creator1/99
  TorqueDemand/100(VTQD_RightSlideRate_pct) -> Bus Creator1/100
  TorqueDemand/101(VTQD_FrontSlideRate_pct) -> Bus Creator1/101
  TorqueDemand/102(VTQD_RearSlideRate_pct) -> Bus Creator1/102
  TorqueDemand/103(VTQD_TrailerDisOPDSta_flg) -> Bus Creator1/103
  TorqueDemand/104(VTQD_ComboKeyPreEn_flg) -> Bus Creator1/104
  TorqueDemand/105(VTQD_ComboKeyEn_flg) -> Bus Creator1/105
  TorqueDemand/106(VTQD_SysMode_enum) -> Bus Creator1/106
  TorqueDemand/107(VTQD_WhlTqCapMotFr_Nm) -> Bus Creator1/107
  TorqueDemand/108(VTQD_WhlTqCapMotRr_Nm) -> Bus Creator1/108
  TorqueDemand/109(VTQD_FrShaftSpd_rpm) -> Bus Creator1/109
  TorqueDemand/110(VTQD_RrShaftSpd_rpm) -> Bus Creator1/110
  Bus Selector8/5 -> TorqueDemand/142(VTQR_RShaftSpdTqLimLow_flg)  "<VTQR_RShaftSpdTqLimLow_flg>"
  Bus Selector8/6 -> TorqueDemand/143(VTQR_RTimerTqLimLow_flg)  "<VTQR_RTimerTqLimLow_flg>"
  Bus Selector8/7 -> TorqueDemand/144(VTQR_FShaftSpdTqLimLow_flg)  "<VTQR_FShaftSpdTqLimLow_flg>"
  Bus Selector8/8 -> TorqueDemand/145(VTQR_FTimerTqLimLow_flg)  "<VTQR_FTimerTqLimLow_flg>"
  Bus Selector6/15 -> TorqueDemand/96(VINP_SWC2RCustomizeSta_flg)  "<VINP_SWC2RCustomizeSta_flg>"
  TorqueDemand/32(VTQD_FrEDUAvailBrkRgnTqV_flg) -> Bus Creator1/32
  TorqueDemand/31(VTQD_FrEDUSpdValid_flg) -> Bus Creator1/31
  TorqueDemand/41(VTQD_FrIdcMax_A) -> Bus Creator1/41
  TorqueDemand/40(VTQD_FrIdcMin_A) -> Bus Creator1/40
  TorqueDemand/39(VTQD_ExternalTqAllow_flg) -> Bus Creator1/39
  TorqueDemand/38(VTQD_RrRgnPermSta_flg) -> Bus Creator1/38
  TorqueDemand/37(VTQD_FrRgnPermSta_flg) -> Bus Creator1/37
  TorqueDemand/36(VTQD_PTCSPermSta_flg) -> Bus Creator1/36
  TorqueDemand/35(VTQD_RgnAbnorSta_flg) -> Bus Creator1/35
  TorqueDemand/34(VTQD_RrEDUAvailBrkRgnTqV_flg) -> Bus Creator1/34
  TorqueDemand/33(VTQD_RrEDUSpdValid_flg) -> Bus Creator1/33
  TorqueDemand/23(VTQD_DriverWhlTqDemFr_Nm) -> Bus Creator1/23
  TorqueDemand/22(VTQD_RrRgnDecrSta_flg) -> Bus Creator1/22
  TorqueDemand/21(VTQD_FrRgnDecrSta_flg) -> Bus Creator1/21
  TorqueDemand/20(VTQD_RrActvDmpDisabReq_flg) -> Bus Creator1/20
  TorqueDemand/19(VTQD_FrActvDmpDisabReq_flg) -> Bus Creator1/19
  TorqueDemand/18(VTQD_PButtonSta_enum) -> Bus Creator1/18
  TorqueDemand/1(VTQD_GearActualPosn_enum) -> Bus Creator1/1
  TorqueDemand/2(VTQD_ParkRequest_flg) -> Bus Creator1/2
  TorqueDemand/3(VTQD_PBWLockTO_flg) -> Bus Creator1/3
  TorqueDemand/4(VTQD_PBWUnlockTO_flg) -> Bus Creator1/4
  TorqueDemand/5(VTQD_DriverWhlTqDem_Nm) -> Bus Creator1/5
  TorqueDemand/6(VTQD_AfterAvailableTqDemFr_Nm) -> Bus Creator1/6
  TorqueDemand/7(VTQD_AfterAvailableTqDemRr_Nm) -> Bus Creator1/7
  TorqueDemand/8(VTQD_TqSourceFr_enum) -> Bus Creator1/8
  TorqueDemand/9(VTQD_TqSourceRr_enum) -> Bus Creator1/9
  TorqueDemand/10(VTQD_FrEDUAvailBrkRgnTq_Nm) -> Bus Creator1/10
  TorqueDemand/11(VTQD_RrEDUAvailBrkRgnTq_Nm) -> Bus Creator1/11
  TorqueDemand/12(VTQD_TqTargetShaftSpd_rpm) -> Bus Creator1/12
  TorqueDemand/13(VTQD_LimpHomeAct_flg) -> Bus Creator1/13
  TorqueDemand/14(VTQD_RollRegenEnable_flg) -> Bus Creator1/14
  TorqueDemand/15(VTQD_EVDriveMode_enum) -> Bus Creator1/15
  TorqueDemand/16(VTQD_EVDriveModeValid_flg) -> Bus Creator1/16
  TorqueDemand/17(VTQD_ShiftGearPosn_enum) -> Bus Creator1/17
  Bus Selector8/9 -> TorqueDemand/146(VTQR_FrFirstOrderInpTs_c)  "<VTQR_FrFirstOrderInpTs_c>"
  Bus Selector8/10 -> TorqueDemand/147(VTQR_RrFirstOrderInpTs_c)  "<VTQR_RrFirstOrderInpTs_c>"
  Bus Selector8/11 -> TorqueDemand/148(VTQR_FrRateLimitInc_Nm)  "<VTQR_FrRateLimitInc_Nm>"
  Bus Selector8/12 -> TorqueDemand/149(VTQR_FrRateLimitDec_Nm)  "<VTQR_FrRateLimitDec_Nm>"
  Bus Selector8/13 -> TorqueDemand/150(VTQR_RrRateLimitInc_Nm)  "<VTQR_RrRateLimitInc_Nm>"
  Bus Selector8/14 -> TorqueDemand/151(VTQR_RrRateLimitDec_Nm)  "<VTQR_RrRateLimitDec_Nm>"
  Bus Selector13/13 -> TorqueDemand/76(VINP_FrMCUDCBusVolt_V)  "<VINP_FrMCUDCBusVolt_V>"
  Bus Selector13/14 -> TorqueDemand/77(VINP_RrMCUDCBusVolt_V)  "<VINP_RrMCUDCBusVolt_V>"
  TorqueDemand/111(VTQD_EPBCarWashMode_flg) -> Bus Creator1/111
  Bus Selector12/2 -> TorqueDemand/166(VINP_APSStaSystem_enum)  "<VINP_APSStaSystem_enum>"
  Bus Selector13/18 -> TorqueDemand/81(VINP_RrTMTemp_C)  "<VINP_RrTMTemp_C>"
  Bus Selector13/17 -> TorqueDemand/80(VINP_RrMCUTemp_C)  "<VINP_RrMCUTemp_C>"
  Bus Selector13/16 -> TorqueDemand/79(VINP_FrTMTemp_C)  "<VINP_FrTMTemp_C>"
  Bus Selector13/15 -> TorqueDemand/78(VINP_FrMCUTemp_C)  "<VINP_FrMCUTemp_C>"
  Bus Selector9/5 -> TorqueDemand/161(VINP_ADASAEBSta_enum)  "<VINP_ADASAEBSta_enum>"
  TorqueDemand/112(VTQD_IVIRockModeEn_flg) -> Bus Creator1/112
  TorqueDemand/116(VTQD_SimSouWaveReq_pct) -> Bus Creator1/116
  Bus Selector2/36 -> TorqueDemand/42(VINP_ESCOFFStatus_enum)  "<VINP_ESCOFFStatus_enum>"
  TorqueDemand/117(VTQD_RockModeTCSReq_flg) -> Bus Creator1/117
  BDDM_outputs/1 -> Bus Selector15/1
  Bus Selector15/2 -> TorqueDemand/170(VDDM_VCURAPSErrLv3_flg)  "<VDDM_VCURAPSErrLv3_flg>"
  Bus Selector15/3 -> TorqueDemand/171(VDDM_EPBSigErrCFS_flg)  "<VDDM_EPBSigErrCFS_flg>"
  Bus Selector15/1 -> TorqueDemand/169(VDDM_VCURAPSErrLv2_flg)  "<VDDM_VCURAPSErrLv2_flg>"
  Bus Selector8/15 -> TorqueDemand/152(VTQR_FrTqZeroTransLowBound_Nm)  "<VTQR_FrTqZeroTransLowBound_Nm>"
  Bus Selector8/16 -> TorqueDemand/153(VTQR_RrTqZeroTransUpBound_Nm)  "<VTQR_RrTqZeroTransUpBound_Nm>"
  TorqueDemand/118(VTQD_TMEnOutpTqSta_enum) -> Bus Creator1/118
  Bus Selector15/4 -> TorqueDemand/172(VDDM_EPB1Err_flg)  "<VDDM_EPB1Err_flg>"
  Bus Selector15/5 -> TorqueDemand/173(VDDM_ESC1Err_flg)  "<VDDM_ESC1Err_flg>"
  Bus Selector15/6 -> TorqueDemand/174(VDDM_ESC5Err_flg)  "<VDDM_ESC5Err_flg>"
  Bus Selector15/7 -> TorqueDemand/175(VDDM_LimpHomeAct_flg)  "<VDDM_LimpHomeAct_flg>"
  Bus Selector15/8 -> TorqueDemand/176(VDDM_VehMalfunLevel_enum)  "<VDDM_VehMalfunLevel_enum>"
  Bus Selector15/9 -> TorqueDemand/177(VDDM_Shifter1Err_flg)  "<VDDM_Shifter1Err_flg>"
  Bus Selector15/10 -> TorqueDemand/178(VDDM_ShifterSigErrCFS_flg)  "<VDDM_ShifterSigErrCFS_flg>"
  Bus Selector15/11 -> TorqueDemand/179(VDDM_MCUF1Err_flg)  "<VDDM_MCUF1Err_flg>"
  Bus Selector15/12 -> TorqueDemand/180(VDDM_MCUR1Err_flg)  "<VDDM_MCUR1Err_flg>"
  Bus Selector15/13 -> TorqueDemand/181(VDDM_RegenErrCFS_flg)  "<VDDM_RegenErrCFS_flg>"
  Bus Selector15/14 -> TorqueDemand/182(VDDM_4D2CErr_flg)  "<VDDM_4D2CErr_flg>"
  Bus Selector4/11 -> TorqueDemand/63(VINP_ShifterFailsta_enum)  "<VINP_ShifterFailsta_enum>"
  TorqueDemand/113(VTQD_ForceP_flg) -> Bus Creator1/113
  TorqueDemand/114(VTQD_SlideRegenLimTq_Nm) -> Bus Creator1/114
  TorqueDemand/115(VTQD_SimSoundCmd_pct) -> Bus Creator1/115

== system tqd/Model Info/EmptySubsystem ==

== system tqd/TQD/SWC_HandShake ==
  In1 : Inport
  Bus Creator : BusCreator  Inputs=2
  Bus Selector : BusSelector  OutputSignals=VINP_SWC2LRegenUpSta_flg,VINP_SWCRegenUp_flg,VINP_SWC2RRegenDownSta_flg,VINP_SWCRegenDown_flg
  Logical Operator : Logic  Operator=OR  AllPortsSameDT=off  OutDataTypeStr=boolean
  Logical Operator1 : Logic  Operator=OR  AllPortsSameDT=off  OutDataTypeStr=boolean
  BTQD_CAN4SWC_outputs : Outport
  wires:
  In1/1 -> Bus Selector/1
  Bus Selector/1 -> Logical Operator/1  "<VINP_SWC2LRegenUpSta_flg>"
  Bus Selector/2 -> Logical Operator/2  "<VINP_SWCRegenUp_flg>"
  Bus Selector/3 -> Logical Operator1/1  "<VINP_SWC2RRegenDownSta_flg>"
  Bus Selector/4 -> Logical Operator1/2  "<VINP_SWCRegenDown_flg>"
  Logical Operator/1 -> Bus Creator/1  "VINP_SWCRegenUp_flg"
  Logical Operator1/1 -> Bus Creator/2  "VINP_SWCRegenDown_flg"
  Bus Creator/1 -> BTQD_CAN4SWC_outputs/1

== system tqd/TQD/Subsystem ==
  BINP_CAN3_outputs : Inport
  Bus Creator : BusCreator  Inputs=18
  Bus Selector1 : BusSelector  OutputSignals=VINP_CANMsgValidMCUNR1_flg,VINP_FrEDURotateDirctionNidec_enum,VINP_FrEDURotateDirction_enum,VINP_RrEDURotateDirctionNidec_enum,VINP_RrEDURotateDirction_enum,VINP_FrTMSpdNidec_rpm,VINP_FrTMSpd_rpm,VINP_RrTMSpdNidec_rpm,VINP_RrTMSpd_rpm,VINP_FrRegenAvailTqNidec_Nm,VINP_FrRegenAvailTq_Nm,VINP_RrRegenAvailTqNidec_Nm,VINP_RrRegenAvailTq_Nm,VINP_FrEDURealTMTqNidec_Nm,VINP_FrEDURealTMTq_Nm,VINP_RrEDURealTMTqNidec_Nm,VINP_RrEDURealTMTq_Nm,VINP_FrMotorAvailTqNidec_Nm,VINP_FrMotorAvailTq_Nm,VINP_RrMotorAvailTqNidec_Nm,VINP_RrMotorAvailTq_Nm,VINP_MCUWarnFNidec_enum,VINP_MCUWarnF_enum,VINP_MCUWarnRNidec_enum,VINP_MCUWarnR_enum,VINP_FrMCUDCBusVoltNidec_V,VINP_FrMCUDCBusVolt_V,VINP_RrMCUDCBusVoltNidec_V,VINP_RrMCUDCBusVolt_V,VINP_FrMCUTempNidec_C,VINP_FrMCUTemp_C,VINP_FrTMTempNidec_C,VINP_FrTMTemp_C,VINP_RrMCUTempNidec_C,VINP_RrMCUTemp_C,VINP_RrTMTempNidec_C,VINP_RrTMTemp_C
  Switch{,1..17} (18 alike) : Switch  Criteria=u2 ~= 0
  BTQD_CAN3MCU_outputs : Outport
  wires:
  BINP_CAN3_outputs/1 -> Bus Selector1/1
  Bus Selector1/1 -> [VINP_CANMsgValidMCUNR1_flg]  "<VINP_CANMsgValidMCUNR1_flg>"
  Bus Selector1/3 -> Switch/3  "<VINP_FrEDURotateDirction_enum>"
  Bus Selector1/2 -> Switch/1  "<VINP_FrEDURotateDirctionNidec_enum>"
  Bus Selector1/5 -> Switch1/3  "<VINP_RrEDURotateDirction_enum>"
  [VINP_CANMsgValidMCUNR1_flg] -> Switch1/2
  [VINP_CANMsgValidMCUNR1_flg] -> Switch/2
  Bus Selector1/4 -> Switch1/1  "<VINP_RrEDURotateDirctionNidec_enum>"
  Bus Selector1/8 -> Switch3/1  "<VINP_RrTMSpdNidec_rpm>"
  [VINP_CANMsgValidMCUNR1_flg] -> Switch2/2
  [VINP_CANMsgValidMCUNR1_flg] -> Switch3/2
  Bus Selector1/9 -> Switch3/3  "<VINP_RrTMSpd_rpm>"
  Bus Selector1/6 -> Switch2/1  "<VINP_FrTMSpdNidec_rpm>"
  Bus Selector1/7 -> Switch2/3  "<VINP_FrTMSpd_rpm>"
  Bus Selector1/15 -> Switch6/3  "<VINP_FrEDURealTMTq_Nm>"
  Bus Selector1/14 -> Switch6/1  "<VINP_FrEDURealTMTqNidec_Nm>"
  Bus Selector1/17 -> Switch7/3  "<VINP_RrEDURealTMTq_Nm>"
  [VINP_CANMsgValidMCUNR1_flg] -> Switch7/2
  [VINP_CANMsgValidMCUNR1_flg] -> Switch6/2
  Bus Selector1/16 -> Switch7/1  "<VINP_RrEDURealTMTqNidec_Nm>"
  Bus Selector1/12 -> Switch5/1  "<VINP_RrRegenAvailTqNidec_Nm>"
  [VINP_CANMsgValidMCUNR1_flg] -> Switch4/2
  [VINP_CANMsgValidMCUNR1_flg] -> Switch5/2
  Bus Selector1/13 -> Switch5/3  "<VINP_RrRegenAvailTq_Nm>"
  Bus Selector1/10 -> Switch4/1  "<VINP_FrRegenAvailTqNidec_Nm>"
  Bus Selector1/11 -> Switch4/3  "<VINP_FrRegenAvailTq_Nm>"
  Bus Selector1/19 -> Switch8/3  "<VINP_FrMotorAvailTq_Nm>"
  Bus Selector1/18 -> Switch8/1  "<VINP_FrMotorAvailTqNidec_Nm>"
  Bus Selector1/21 -> Switch9/3  "<VINP_RrMotorAvailTq_Nm>"
  [VINP_CANMsgValidMCUNR1_flg] -> Switch9/2
  [VINP_CANMsgValidMCUNR1_flg] -> Switch8/2
  Bus Selector1/20 -> Switch9/1  "<VINP_RrMotorAvailTqNidec_Nm>"
  Bus Selector1/24 -> Switch11/1  "<VINP_MCUWarnRNidec_enum>"
  [VINP_CANMsgValidMCUNR1_flg] -> Switch10/2
  [VINP_CANMsgValidMCUNR1_flg] -> Switch11/2
  Bus Selector1/25 -> Switch11/3  "<VINP_MCUWarnR_enum>"
  Bus Selector1/22 -> Switch10/1  "<VINP_MCUWarnFNidec_enum>"
  Bus Selector1/23 -> Switch10/3  "<VINP_MCUWarnF_enum>"
  Switch/1 -> Bus Creator/1  "VINP_FrEDURotateDirction_enum"
  Switch1/1 -> Bus Creator/2  "VINP_RrEDURotateDirction_enum"
  Switch2/1 -> Bus Creator/3  "VINP_FrTMSpd_rpm"
  Switch3/1 -> Bus Creator/4  "VINP_RrTMSpd_rpm"
  Switch4/1 -> Bus Creator/5  "VINP_FrRegenAvailTq_Nm"
  Switch5/1 -> Bus Creator/6  "VINP_RrRegenAvailTq_Nm"
  Switch6/1 -> Bus Creator/7  "VINP_FrEDURealTMTq_Nm"
  Switch7/1 -> Bus Creator/8  "VINP_RrEDURealTMTq_Nm"
  Switch8/1 -> Bus Creator/9  "VINP_FrMotorAvailTq_Nm"
  Switch9/1 -> Bus Creator/10  "VINP_RrMotorAvailTq_Nm"
  Switch10/1 -> Bus Creator/11  "VINP_MCUWarnF_enum"
  Switch11/1 -> Bus Creator/12  "VINP_MCUWarnR_enum"
  Bus Creator/1 -> BTQD_CAN3MCU_outputs/1
  [VINP_CANMsgValidMCUNR1_flg] -> Switch12/2
  [VINP_CANMsgValidMCUNR1_flg] -> Switch13/2
  Bus Selector1/27 -> Switch12/3  "<VINP_FrMCUDCBusVolt_V>"
  Bus Selector1/26 -> Switch12/1  "<VINP_FrMCUDCBusVoltNidec_V>"
  Bus Selector1/28 -> Switch13/1  "<VINP_RrMCUDCBusVoltNidec_V>"
  Bus Selector1/29 -> Switch13/3  "<VINP_RrMCUDCBusVolt_V>"
  Switch12/1 -> Bus Creator/13  "VINP_FrMCUDCBusVolt_V"
  Switch13/1 -> Bus Creator/14  "VINP_RrMCUDCBusVolt_V"
  [VINP_CANMsgValidMCUNR1_flg] -> Switch14/2
  Bus Selector1/30 -> Switch14/1  "<VINP_FrMCUTempNidec_C>"
  Bus Selector1/31 -> Switch14/3  "<VINP_FrMCUTemp_C>"
  [VINP_CANMsgValidMCUNR1_flg] -> Switch15/2
  Bus Selector1/32 -> Switch15/1  "<VINP_FrTMTempNidec_C>"
  Bus Selector1/33 -> Switch15/3  "<VINP_FrTMTemp_C>"
  Bus Selector1/35 -> Switch16/3  "<VINP_RrMCUTemp_C>"
  [VINP_CANMsgValidMCUNR1_flg] -> Switch16/2
  Bus Selector1/34 -> Switch16/1  "<VINP_RrMCUTempNidec_C>"
  Bus Selector1/36 -> Switch17/1  "<VINP_RrTMTempNidec_C>"
  Bus Selector1/37 -> Switch17/3  "<VINP_RrTMTemp_C>"
  Switch14/1 -> Bus Creator/15  "VINP_FrMCUTemp_C"
  Switch15/1 -> Bus Creator/16  "VINP_FrTMTemp_C"
  Switch16/1 -> Bus Creator/17  "VINP_RrMCUTemp_C"
  Switch17/1 -> Bus Creator/18  "VINP_RrTMTemp_C"
  [VINP_CANMsgValidMCUNR1_flg] -> Switch17/2
